simulink model "task123"  (R2019b)
settings: Solver=VariableStepAuto  StartTime=0.0  StopTime=10.0  RelTol=1e-3
values from neighbouring files (symbols this model uses):
  yd1 = c2d(y,ds1)    [plant_descretization.m]
  yd2 = c2d(y,ds2)    [plant_descretization.m]
  yd3 = c2d(y,ds3)    [plant_descretization.m]
settings Model: Creator=е  LastModifiedBy=Eugene
settings DebuggingCC: ArithmeticOperatorsInVariantConditions=warning
settings SFSimCC: CustomCodeUndefinedFunction=UseInterfaceOnly

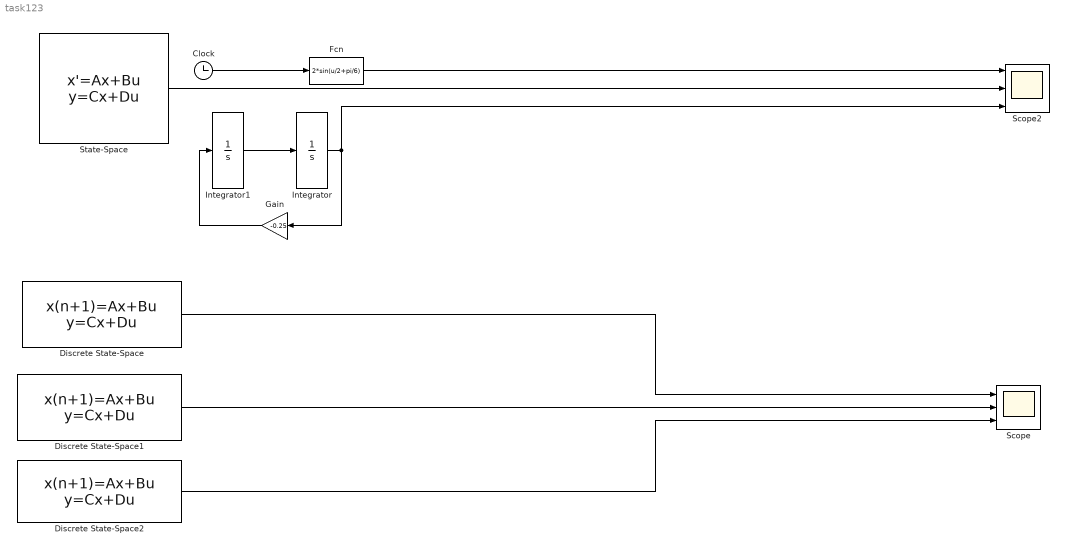
== system task123 ==
  Clock : Clock
  Discrete State-Space : DiscreteStateSpace  A=yd1.A  B=yd1.B  C=yd1.C  D=yd1.D  InitialCondition=[2*sin(pi/6) cos(pi/6)]  SampleTime=0.2
  Discrete State-Space1 : DiscreteStateSpace  A=yd2.A  B=yd2.B  C=yd2.C  D=yd2.D  InitialCondition=[2*sin(pi/6) cos(pi/6)]  SampleTime=0.02
  Discrete State-Space2 : DiscreteStateSpace  A=yd3.A  B=yd3.B  C=yd3.C  D=yd3.D  InitialCondition=[2*sin(pi/6) cos(pi/6)]  SampleTime=0.002
  Fcn : Fcn  Expr=2*sin(u/2+pi/6)
  Gain : Gain  Gain=-0.25
  Integrator : Integrator  InitialCondition=2*sin(pi/6)  ContinuousStateAttributes='position'
  Integrator1 : Integrator  InitialCondition=cos(pi/6)  ContinuousStateAttributes='position'
  Scope : Scope  NumInputPorts=3
  Scope2 : Scope  NumInputPorts=3
  State-Space : StateSpace  A=[0 1; -0.25 0]  B=[0; 0]  C=[1 0]  D=0  InitialCondition=[2*sin(pi/6) cos(pi/6)]  ContinuousStateAttributes='position'
  wires:
  Gain/1 -> Integrator1/1
  Integrator1/1 -> Integrator/1
  Clock/1 -> Fcn/1
  Fcn/1 -> Scope2/1
  State-Space/1 -> Scope2/2
  Discrete State-Space/1 -> Scope/1
  Discrete State-Space1/1 -> Scope/2
  Discrete State-Space2/1 -> Scope/3
  Integrator/1 -> Scope2/3, Gain/1
